simulink subsystem "PowerGain"  (R2022b)
settings: Solver=VariableStepAuto  StartTime=0.0  StopTime=10.0  RelTol=1e-3
undefined symbols (not defined in the file): ProjectExample, T_power
settings Model: Creator=Ilya_Andriyanov  LastModifiedBy=user

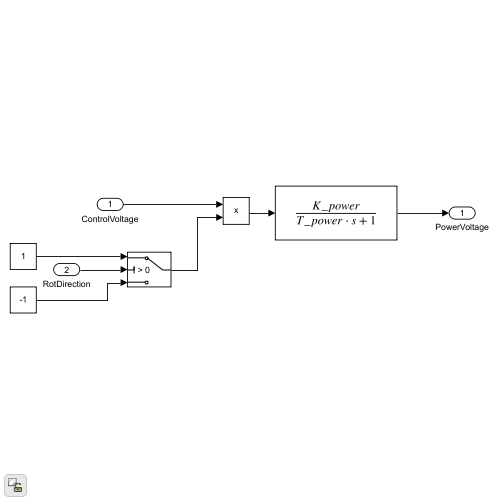
[thumbnail: Simulink's stored preview of the top-level diagram]
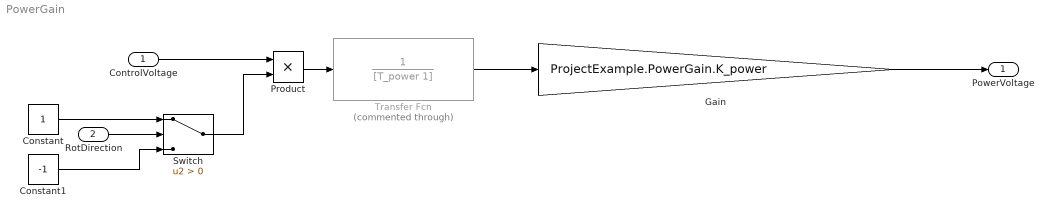
== system PowerGain ==
  ControlVoltage : Inport
  RotDirection : Inport  Port=2
  Constant : Constant
  Constant1 : Constant  Value=-1
  Gain : Gain  Gain=ProjectExample.PowerGain.K_power
  Product : Product
  Switch : Switch  Criteria=u2 > Threshold  SaturateOnIntegerOverflow=off  InputSameDT=off
  Transfer Fcn : TransferFcn  Commented=through  Denominator=[T_power 1]
  PowerVoltage : Outport
  wires:
  Transfer Fcn/1 -> Gain/1
  RotDirection/1 -> Switch/2
  Constant/1 -> Switch/1
  Constant1/1 -> Switch/3
  Product/1 -> Transfer Fcn/1
  ControlVoltage/1 -> Product/1
  Switch/1 -> Product/2
  Gain/1 -> PowerVoltage/1
